simulink model "MADKAL"  (R2015a)
settings: Solver=ode45  StartTime=0.0  StopTime=10.0  RelTol=1e-3
values from neighbouring files (symbols this model uses):
  ba_e = zeros(3,1)    [Parameters.m]
  bb_e = 0    [Parameters.m]
  bg_e = zeros(3,1)    [Parameters.m]
  bm_e = zeros(3,1)    [Parameters.m]
  Ex = zeros(10,1)    [Parameters.m]
  g = 9.81    [Parameters.m]
  g_e = g    (= 9.81)    [Parameters.m]
  G_e = eye(3)    [Parameters.m]
  Ix_e = Ixx    (= 0.034736)    [Parameters.m]
  Iy_e = Iyy    (= 0.034736)    [Parameters.m]
  Iz_e = Izz    (= 0.069472)    [Parameters.m]
  kb_e = 1    [Parameters.m]
  m_e = m    (= 1.478)    [Parameters.m]
  Ma_e = eye(3)    [Parameters.m]
  mag_field = mag / norm(mag)    [Parameters.m]
  mf_e = mf_e /norm(mf_e)    [Parameters.m]
  Mg_e = eye(3)    [Parameters.m]
  P0 = 101325    [Parameters.m]
  P0_e = P0    (= 101325)    [Parameters.m]
  Q_e = 0.005*eye(10)    [Parameters.m]
  R_e = [ 0.0001   0 0 0 0 0 0 0 0 0 ... (first row only)    [Parameters.m]
  Ra = 286.9    [Parameters.m]
  Ra_e = Ra    (= 286.9)    [Parameters.m]
  T0 = 293.15    [Parameters.m]
  T0_e = T0    (= 293.15)    [Parameters.m]
  Ts = 1/200    (= 0.005)    [Parameters.m]
  Varx = 0.001*eye(10)    [Parameters.m]
undefined symbols (not defined in the file or in its folder): freqMadgwick, gain_aa, poles_aa, zeros_aa
libraries: Quadrotor_tools x16, simulink x1, simulink_extras x1
(part 1 of 2)
settings Model: Creator=Mattia  LastModifiedBy=Mattia

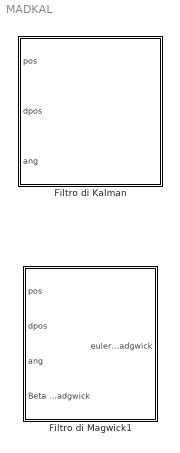
== system MADKAL ==
  Filtro di Kalman : Subsystem
  Filtro di Magwick1 : Subsystem

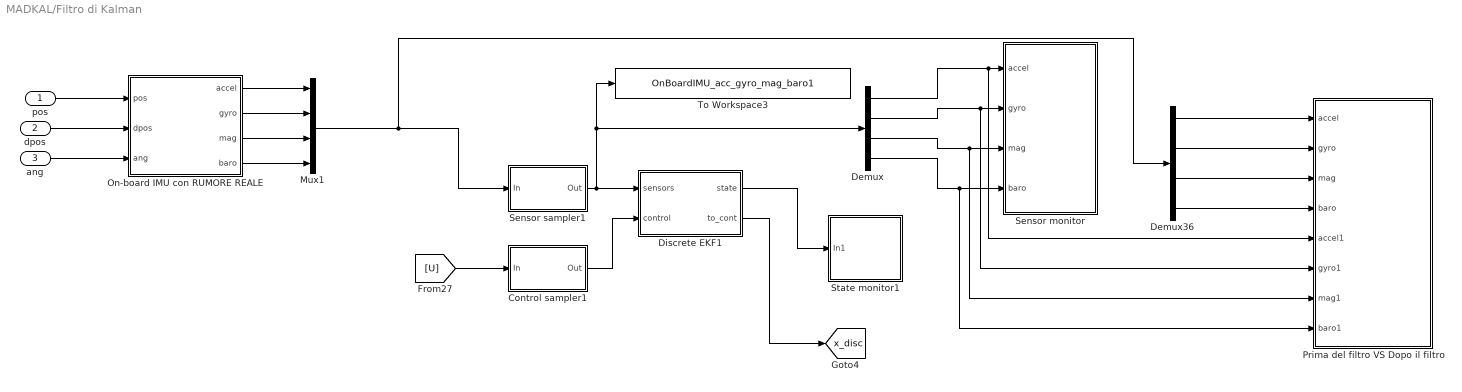
== system MADKAL/Filtro di Kalman ==
  pos : Inport
  dpos : Inport  Port=2
  ang : Inport  Port=3
  Control sampler1 : Subsystem
  Demux : Demux  Outputs=[3 3 3 1]
  Demux36 : Demux  Outputs=[3 3 3 1]
  Discrete EKF1 : Subsystem
  Mux1 : Mux
  On-board IMU con RUMORE REALE : Subsystem
  Prima del filtro VS Dopo il filtro : Subsystem
  Sensor monitor : Subsystem
  Sensor sampler1 : Subsystem
  State monitor1 : Subsystem
  To Workspace3 : ToWorkspace  VariableName=OnBoardIMU_acc_gyro_mag_baro1  SaveFormat=Timeseries  SampleTime=-1
  tag scope: x_disc=global
  wires:
  Demux36/4 -> Prima del filtro VS Dopo il filtro/4(baro)
  Demux36/1 -> Prima del filtro VS Dopo il filtro/1(accel)
  Demux36/2 -> Prima del filtro VS Dopo il filtro/2(gyro)
  Demux36/3 -> Prima del filtro VS Dopo il filtro/3(mag)
  Sensor sampler1/1(Out) -> Discrete EKF1/1(sensors), Demux/1, To Workspace3/1
  [U] -> Control sampler1/1(In)
  Control sampler1/1(Out) -> Discrete EKF1/2(control)
  Demux/1 -> Prima del filtro VS Dopo il filtro/5(accel1), Sensor monitor/1(accel)
  Demux/2 -> Prima del filtro VS Dopo il filtro/6(gyro1), Sensor monitor/2(gyro)
  On-board IMU con RUMORE REALE/1(accel) -> Mux1/1
  Demux/3 -> Prima del filtro VS Dopo il filtro/7(mag1), Sensor monitor/3(mag)
  On-board IMU con RUMORE REALE/4(baro) -> Mux1/4
  On-board IMU con RUMORE REALE/3(mag) -> Mux1/3
  On-board IMU con RUMORE REALE/2(gyro) -> Mux1/2
  Demux/4 -> Prima del filtro VS Dopo il filtro/8(baro1), Sensor monitor/4(baro)
  dpos/1 -> On-board IMU con RUMORE REALE/2(dpos)
  pos/1 -> On-board IMU con RUMORE REALE/1(pos)
  ang/1 -> On-board IMU con RUMORE REALE/3(ang)
  Discrete EKF1/1(state) -> State monitor1/1(In1)
  Discrete EKF1/2("to_cont ") -> [x_disc]
  Mux1/1 -> Sensor sampler1/1(In), Demux36/1

== system MADKAL/Filtro di Magwick1 ==
  pos : Inport
  dpos : Inport  Port=2
  ang : Inport  Port=3
  Beta Madgwick : Inport  Port=4
  Demux11 : Demux  Outputs=[3 3 3 1]
  Madgwickcodice OK2 : Subsystem
  Mux10 : Mux
  On-board IMUcon RUMORE REALE : Subsystem
  Sensor monitor1 : Subsystem
  To Workspace1 : ToWorkspace  VariableName=OnBoardIMU_acc_gyro_mag_baroXX  SaveFormat=Timeseries  SampleTime=-1
  eulero Madgwick : Outport
  wires:
  pos/1 -> On-board IMUcon RUMORE REALE/1(pos)
  ang/1 -> On-board IMUcon RUMORE REALE/3(ang)
  dpos/1 -> On-board IMUcon RUMORE REALE/2(dpos)
  Demux11/4 -> Sensor monitor1/4(baro)
  Demux11/2 -> Sensor monitor1/2(gyro)
  On-board IMUcon RUMORE REALE/1(accel) -> Mux10/1
  Demux11/1 -> Sensor monitor1/1(accel)
  On-board IMUcon RUMORE REALE/3(mag) -> Mux10/3
  On-board IMUcon RUMORE REALE/2(gyro) -> Mux10/2
  Demux11/3 -> Sensor monitor1/3(mag)
  On-board IMUcon RUMORE REALE/4(baro) -> Mux10/4
  Beta Madgwick/1 -> Madgwickcodice OK2/2(Beta Madgwick)
  Madgwickcodice OK2/1(eulerMadgwick) -> eulero Madgwick/1
  Mux10/1 -> To Workspace1/1, Demux11/1, Madgwickcodice OK2/1(In)

== system MADKAL/Filtro di Kalman/Control sampler1 ==
  In : Inport
  Anti-aliasing : Subsystem
  Rate Transition : RateTransition  OutPortSampleTime=Ts
  Out : Outport
  wires:
  Anti-aliasing/1(Out1) -> Rate Transition/1
  In/1 -> Anti-aliasing/1(In1)
  Rate Transition/1 -> Out/1

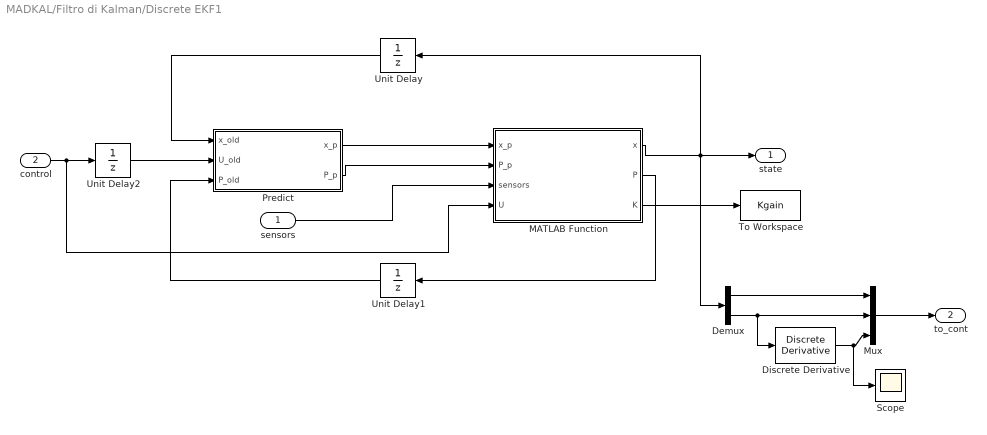
== system MADKAL/Filtro di Kalman/Discrete EKF1 ==
  sensors : Inport
  control : Inport  Port=2
  Demux : Demux  Outputs=[9 1]
  Discrete Derivative : simulink/Discrete/Discrete Derivative  gainval=1.0  ICPrevScaledInput=0.0  InputProcessing=Inherited  OutMin=[]  OutMax=[]  OutDataType=fixdt(1, 16)  OutScaling=2^-10  DoSatur=off
  MATLAB Function : MATLAB Function  TreatAsAtomicUnit=on
  Mux : Mux  Inputs=3
  "Predict " : MATLAB Function  TreatAsAtomicUnit=on
  Scope : Scope
      settings: SaveName=ScopeData20
  To Workspace : ToWorkspace  VariableName=Kgain  SaveFormat=Timeseries  SampleTime=-1
  Unit Delay : UnitDelay  InitialCondition=Ex  SampleTime=Ts
  Unit Delay1 : UnitDelay  InitialCondition=Varx  SampleTime=Ts
  Unit Delay2 : UnitDelay  InitialCondition=[g_e*m_e; 0; 0; 0]  SampleTime=Ts
  state : Outport
  "to_cont " : Outport  Port=2
  wires:
  "Predict "/2(P_p) -> MATLAB Function/2(P_p)
  sensors/1 -> MATLAB Function/3(sensors)
  MATLAB Function/1(x) -> Demux/1, state/1, Unit Delay/1
  Unit Delay/1 -> "Predict "/1(x_old)
  MATLAB Function/2(P) -> Unit Delay1/1
  Unit Delay1/1 -> "Predict "/3(P_old)
  control/1 -> MATLAB Function/4(U), Unit Delay2/1
  Unit Delay2/1 -> "Predict "/2(U_old)
  "Predict "/1(x_p) -> MATLAB Function/1(x_p)
  MATLAB Function/3(K) -> To Workspace/1
  Demux/1 -> Mux/1
  Mux/1 -> "to_cont "/1
  Demux/2 -> Discrete Derivative/1, Mux/2
  Discrete Derivative/1 -> Scope/1, Mux/3

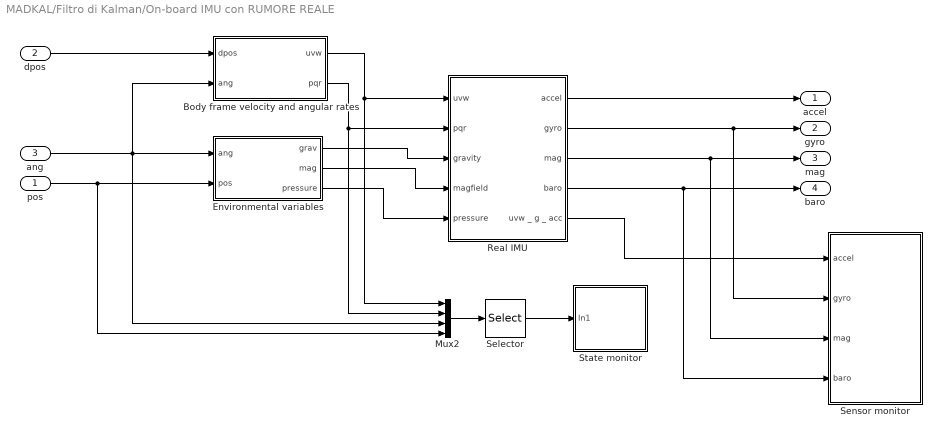
== system MADKAL/Filtro di Kalman/On-board IMU con RUMORE REALE ==
  pos : Inport
  dpos : Inport  Port=2
  ang : Inport  Port=3
  Body frame velocity and angular rates : Subsystem
  Environmental variables : Subsystem
  Mux2 : Mux
  Real IMU : Subsystem
  Selector : Selector  InputPortWidth=12  Indices=[1 2 3 4 5 6 7 8 9 12]
  Sensor monitor : Subsystem
  State monitor : Subsystem
  accel : Outport
  gyro : Outport  Port=2
  mag : Outport  Port=3
  baro : Outport  Port=4
  wires:
  Body frame velocity and angular rates/2(pqr) -> Mux2/2, Real IMU/2(pqr)
  Body frame velocity and angular rates/1(uvw) -> Mux2/1, Real IMU/1(uvw)
  Environmental variables/1(grav) -> Real IMU/3(gravity)
  Environmental variables/2(mag) -> Real IMU/4(magfield)
  Environmental variables/3(pressure) -> Real IMU/5(pressure)
  Mux2/1 -> Selector/1
  Selector/1 -> State monitor/1(In1)
  Real IMU/4(baro) -> Sensor monitor/4(baro), baro/1
  Real IMU/3(mag) -> Sensor monitor/3(mag), mag/1
  Real IMU/2(gyro) -> gyro/1, Sensor monitor/2(gyro)
  Real IMU/1(accel) -> accel/1
  pos/1 -> Mux2/4, Environmental variables/2(pos)
  dpos/1 -> Body frame velocity and angular rates/1(dpos)
  ang/1 -> Body frame velocity and angular rates/2(ang), Mux2/3, Environmental variables/1(ang)
  Real IMU/5(uvw _ g _ acc) -> Sensor monitor/1(accel)

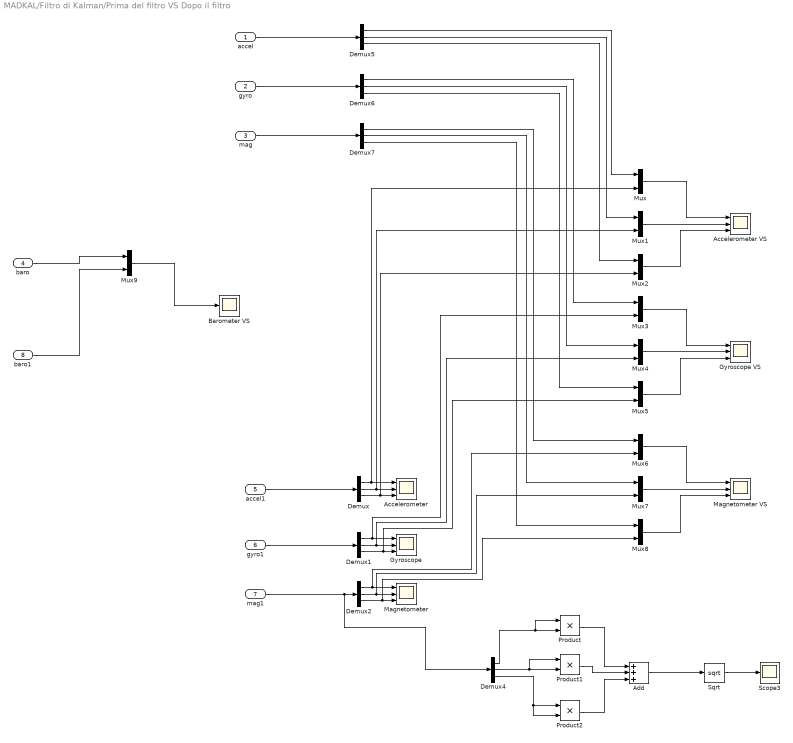
== system MADKAL/Filtro di Kalman/Prima del filtro VS Dopo il filtro ==
  accel : Inport
  gyro : Inport  Port=2
  mag : Inport  Port=3
  baro : Inport  Port=4
  accel1 : Inport  Port=5
  gyro1 : Inport  Port=6
  mag1 : Inport  Port=7
  baro1 : Inport  Port=8
  Accelerometer : Scope  NumInputPorts=3
      settings: YMin=-0.45~-0.4~9.35  YMax=0.4~0.45~10.25  SaveName=ScopeData16
  Accelerometer VS : Scope  NumInputPorts=3
      settings: YMin=-0.45~-0.4~9.35  YMax=0.4~0.45~10.25  SaveName=ScopeData110
  Add : Sum  Inputs=+++
  Barometer VS : Scope
      settings: YMin=-0.45  YMax=0.4  SaveName=ScopeData113
  Demux{,1..2,4..7} (7 alike) : Demux  Outputs=3
  Gyroscope : Scope  NumInputPorts=3
      settings: YMin=-5~-5~-5  YMax=5~5~5  SaveName=ScopeData17
  Gyroscope VS : Scope  NumInputPorts=3
      settings: YMin=-0.45~-0.4~9.35  YMax=0.4~0.45~10.25  SaveName=ScopeData111
  Magnetometer : Scope  NumInputPorts=3
      settings: YMin=-5~-5~-5  YMax=5~5~5  SaveName=ScopeData18
  Magnetometer VS : Scope  NumInputPorts=3
      settings: YMin=-0.45~-0.4~9.35  YMax=0.4~0.45~10.25  SaveName=ScopeData112
  Mux{,1..9} (10 alike) : Mux  Inputs=2
  Product : Product
  Product1 : Product
  Product2 : Product
  Scope3 : Scope
      settings: SaveName=ScopeData103
  Sqrt : Sqrt  SaturateOnIntegerOverflow=on
  wires:
  Demux/3 -> Mux2/2, Accelerometer/3
  Demux/2 -> Mux1/2, Accelerometer/2
  Demux/1 -> Mux/2, Accelerometer/1
  accel1/1 -> Demux/1
  Demux1/3 -> Mux5/2, Gyroscope/3
  Demux1/2 -> Mux4/2, Gyroscope/2
  Demux1/1 -> Mux3/2, Gyroscope/1
  gyro1/1 -> Demux1/1
  Demux2/3 -> Mux8/2, Magnetometer/3
  Demux2/2 -> Mux7/2, Magnetometer/2
  Demux2/1 -> Mux6/2, Magnetometer/1
  mag1/1 -> Demux4/1, Demux2/1
  Demux4/3 -> Product2/2, Product2/1
  Demux4/2 -> Product1/2, Product1/1
  Demux4/1 -> Product/2, Product/1
  Product/1 -> Add/1
  Product1/1 -> Add/2
  Product2/1 -> Add/3
  Add/1 -> Sqrt/1
  Sqrt/1 -> Scope3/1
  Demux5/3 -> Mux2/1
  Demux5/2 -> Mux1/1
  Mux/1 -> Accelerometer VS/1
  Mux1/1 -> Accelerometer VS/2
  Mux2/1 -> Accelerometer VS/3
  Mux3/1 -> Gyroscope VS/1
  Mux4/1 -> Gyroscope VS/2
  Mux5/1 -> Gyroscope VS/3
  Mux6/1 -> Magnetometer VS/1
  Mux7/1 -> Magnetometer VS/2
  Mux8/1 -> Magnetometer VS/3
  Demux5/1 -> Mux/1
  Demux6/1 -> Mux3/1
  Demux6/2 -> Mux4/1
  Demux6/3 -> Mux5/1
  Demux7/1 -> Mux6/1
  Demux7/2 -> Mux7/1
  Demux7/3 -> Mux8/1
  accel/1 -> Demux5/1
  gyro/1 -> Demux6/1
  mag/1 -> Demux7/1
  Mux9/1 -> Barometer VS/1
  baro/1 -> Mux9/1
  baro1/1 -> Mux9/2

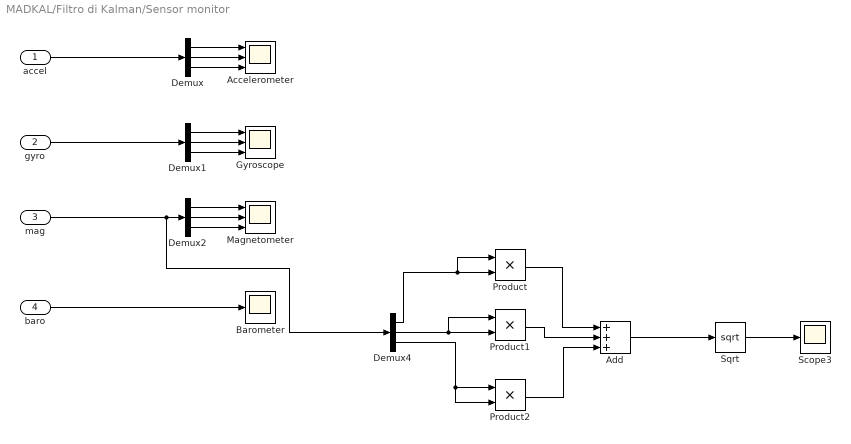
== system MADKAL/Filtro di Kalman/Sensor monitor ==
  accel : Inport
  gyro : Inport  Port=2
  mag : Inport  Port=3
  baro : Inport  Port=4
  Accelerometer : Scope  NumInputPorts=3
      settings: YMin=-0.45~-0.4~9.35  YMax=0.4~0.45~10.25  SaveName=ScopeData16
  Add : Sum  Inputs=+++
  Barometer : Scope
      settings: SaveName=ScopeData19
  Demux{,1..2,4} (4 alike) : Demux  Outputs=3
  Gyroscope : Scope  NumInputPorts=3
      settings: YMin=-5~-5~-5  YMax=5~5~5  SaveName=ScopeData17
  Magnetometer : Scope  NumInputPorts=3
      settings: YMin=-5~-5~-5  YMax=5~5~5  SaveName=ScopeData18
  Product : Product
  Product1 : Product
  Product2 : Product
  Scope3 : Scope
      settings: SaveName=ScopeData103
  Sqrt : Sqrt  SaturateOnIntegerOverflow=on
  wires:
  Demux/3 -> Accelerometer/3
  Demux/2 -> Accelerometer/2
  Demux/1 -> Accelerometer/1
  accel/1 -> Demux/1
  Demux1/3 -> Gyroscope/3
  Demux1/2 -> Gyroscope/2
  Demux1/1 -> Gyroscope/1
  gyro/1 -> Demux1/1
  Demux2/3 -> Magnetometer/3
  Demux2/2 -> Magnetometer/2
  Demux2/1 -> Magnetometer/1
  mag/1 -> Demux4/1, Demux2/1
  baro/1 -> Barometer/1
  Demux4/3 -> Product2/2, Product2/1
  Demux4/2 -> Product1/2, Product1/1
  Demux4/1 -> Product/2, Product/1
  Product/1 -> Add/1
  Product1/1 -> Add/2
  Product2/1 -> Add/3
  Add/1 -> Sqrt/1
  Sqrt/1 -> Scope3/1

== system MADKAL/Filtro di Kalman/Sensor sampler1 ==
  In : Inport
  Anti-aliasing : Subsystem
  Rate Transition : RateTransition  OutPortSampleTime=Ts
  Out : Outport
  wires:
  Rate Transition/1 -> Out/1
  In/1 -> Anti-aliasing/1(In)
  Anti-aliasing/1(Out) -> Rate Transition/1

== system MADKAL/Filtro di Kalman/State monitor1 ==
  In1 : Inport
  Altitude : Scope
      settings: SaveName=ScopeData4
  Angular position : Scope  NumInputPorts=3
      settings: YMin=-5~-5~-5  YMax=5~5~5  SaveName=ScopeData15
  Angular velocity : Scope  NumInputPorts=3
      settings: YMin=-5~-5~-5  YMax=5~5~5  SaveName=ScopeData14
  Demux : Demux  Outputs=[3 3 3 1]
  Demux1 : Demux  Outputs=3
  Demux2 : Demux  Outputs=3
  Demux3 : Demux  Outputs=3
  Linear velocity : Scope  NumInputPorts=3
      settings: YMin=-5~-5~-5  YMax=5~5~5  SaveName=ScopeData13
  To Workspace : ToWorkspace  VariableName=EKFdiscreto_RollPitchYaw  SaveFormat=Timeseries  SampleTime=-1
  tag scope: angKFdisc=global
  wires:
  In1/1 -> Demux/1
  Demux/4 -> Altitude/1
  Demux/1 -> Demux1/1
  Demux1/3 -> Linear velocity/3
  Demux1/2 -> Linear velocity/2
  Demux1/1 -> Linear velocity/1
  Demux/2 -> Demux2/1
  Demux2/3 -> Angular velocity/3
  Demux2/2 -> Angular velocity/2
  Demux2/1 -> Angular velocity/1
  Demux/3 -> [angKFdisc], To Workspace/1, Demux3/1
  Demux3/3 -> Angular position/3
  Demux3/2 -> Angular position/2
  Demux3/1 -> Angular position/1

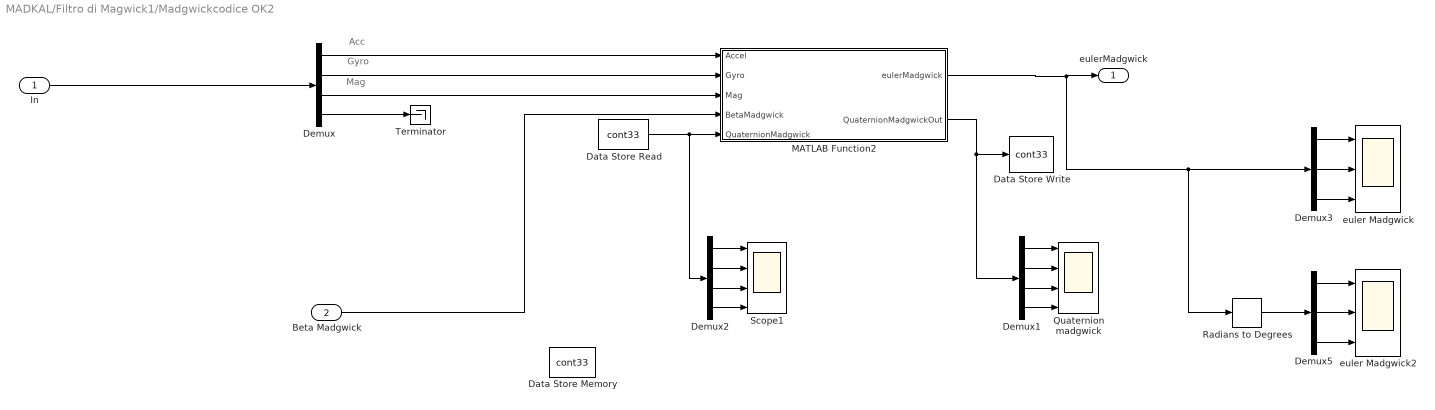
== system MADKAL/Filtro di Magwick1/Madgwickcodice OK2 ==
  note: Mag
  note: Gyro
  note: Acc
  In : Inport
  Beta Madgwick : Inport  Port=2
  Data Store Memory : DataStoreMemory  DataStoreName=cont33  ReadBeforeWriteMsg=warning  WriteAfterWriteMsg=warning  WriteAfterReadMsg=warning  InitialValue=[1 0 0 0]
  Data Store Read : DataStoreRead  DataStoreName=cont33
  Data Store Write : DataStoreWrite  DataStoreName=cont33
  Demux : Demux  Outputs=[3 3 3 1]
  Demux1 : Demux
  Demux2 : Demux
  Demux3 : Demux  Outputs=3
  Demux5 : Demux  Outputs=3
  MATLAB Function2 : MATLAB Function  TreatAsAtomicUnit=on
  Quaternion madgwick : Scope  NumInputPorts=4
      settings: YMin=-5~-5~-5~-5  YMax=5~5~5~5  SaveName=ScopeData89
  Radians to Degrees : simulink_extras/Transformations/Radians to Degrees
  Scope1 : Scope  NumInputPorts=4
      settings: YMin=-5~-5~-5~-5  YMax=5~5~5~5  SaveName=ScopeData90
  Terminator : Terminator
  euler Madgwick : Scope  NumInputPorts=3
      settings: YMin=-5~-5~-5  YMax=5~5~5  SaveName=ScopeData91
  euler Madgwick2 : Scope  NumInputPorts=3
      settings: TimeRange=50  YMin=-5~-5~-5  YMax=5~5~5  SaveName=ScopeData94
  eulerMadgwick : Outport
  wires:
  In/1 -> Demux/1
  Demux/1 -> MATLAB Function2/1(Accel)
  Demux/4 -> Terminator/1
  Demux/3 -> MATLAB Function2/3(Mag)
  Demux/2 -> MATLAB Function2/2(Gyro)
  Data Store Read/1 -> Demux2/1, MATLAB Function2/5(QuaternionMadgwick)
  MATLAB Function2/2(QuaternionMadgwickOut) -> Demux1/1, Data Store Write/1
  Demux1/3 -> Quaternion madgwick/3
  Demux1/4 -> Quaternion madgwick/4
  Demux1/2 -> Quaternion madgwick/2
  Demux1/1 -> Quaternion madgwick/1
  Demux2/3 -> Scope1/3
  Demux2/1 -> Scope1/1
  Demux2/2 -> Scope1/2
  Demux2/4 -> Scope1/4
  Demux3/3 -> euler Madgwick/3
  Demux3/2 -> euler Madgwick/2
  Demux3/1 -> euler Madgwick/1
  Demux5/3 -> euler Madgwick2/3
  Demux5/2 -> euler Madgwick2/2
  Demux5/1 -> euler Madgwick2/1
  Radians to Degrees/1 -> Demux5/1
  Beta Madgwick/1 -> MATLAB Function2/4(BetaMadgwick)
  MATLAB Function2/1(eulerMadgwick) -> Radians to Degrees/1, Demux3/1, eulerMadgwick/1

== system MADKAL/Filtro di Magwick1/On-board IMUcon RUMORE REALE ==
  pos : Inport
  dpos : Inport  Port=2
  ang : Inport  Port=3
  Body frame velocity and angular rates : Subsystem
  Environmental variables : Subsystem
  Mux2 : Mux
  Real IMU : Subsystem
  Selector : Selector  InputPortWidth=12  Indices=[1 2 3 4 5 6 7 8 9 12]
  Sensor monitor : Subsystem
  State monitor : Subsystem
  accel : Outport
  gyro : Outport  Port=2
  mag : Outport  Port=3
  baro : Outport  Port=4
  wires:
  Body frame velocity and angular rates/2(pqr) -> Mux2/2, Real IMU/2(pqr)
  Body frame velocity and angular rates/1(uvw) -> Mux2/1, Real IMU/1(uvw)
  Environmental variables/1(grav) -> Real IMU/3(gravity)
  Environmental variables/2(mag) -> Real IMU/4(magfield)
  Environmental variables/3(pressure) -> Real IMU/5(pressure)
  Mux2/1 -> Selector/1
  Selector/1 -> State monitor/1(In1)
  Real IMU/4(baro) -> Sensor monitor/4(baro), baro/1
  Real IMU/3(mag) -> Sensor monitor/3(mag), mag/1
  Real IMU/2(gyro) -> gyro/1, Sensor monitor/2(gyro)
  Real IMU/1(accel) -> accel/1
  pos/1 -> Mux2/4, Environmental variables/2(pos)
  dpos/1 -> Body frame velocity and angular rates/1(dpos)
  ang/1 -> Body frame velocity and angular rates/2(ang), Mux2/3, Environmental variables/1(ang)
  Real IMU/5(uvw _ g _ acc) -> Sensor monitor/1(accel)

== system MADKAL/Filtro di Magwick1/Sensor monitor1 ==
  accel : Inport
  gyro : Inport  Port=2
  mag : Inport  Port=3
  baro : Inport  Port=4
  Accelerometer : Scope  NumInputPorts=3
      settings: YMin=-5~-5~-5  YMax=5~5~5  SaveName=ScopeData16
  Barometer : Scope
      settings: SaveName=ScopeData19
  Demux : Demux  Outputs=3
  Demux1 : Demux  Outputs=3
  Demux2 : Demux  Outputs=3
  Gyroscope : Scope  NumInputPorts=3
      settings: YMin=-5~-5~-5  YMax=5~5~5  SaveName=ScopeData17
  Magnetometer : Scope  NumInputPorts=3
      settings: YMin=-5~-5~-5  YMax=5~5~5  SaveName=ScopeData18
  wires:
  Demux/3 -> Accelerometer/3
  Demux/2 -> Accelerometer/2
  Demux/1 -> Accelerometer/1
  accel/1 -> Demux/1
  Demux1/3 -> Gyroscope/3
  Demux1/2 -> Gyroscope/2
  Demux1/1 -> Gyroscope/1
  gyro/1 -> Demux1/1
  Demux2/3 -> Magnetometer/3
  Demux2/2 -> Magnetometer/2
  Demux2/1 -> Magnetometer/1
  mag/1 -> Demux2/1
  baro/1 -> Barometer/1

== system MADKAL/Filtro di Kalman/Control sampler1/Anti-aliasing ==
  In1 : Inport
  Bias : Bias  Bias=-g_e*m_e
  Bias1 : Bias  Bias=+g_e*m_e
  Demux : Demux
  Mux : Mux
  Zero-Pole{,1..3} (4 alike) : ZeroPole  Zeros=zeros_aa  Poles=poles_aa  Gain=gain_aa
  Out1 : Outport
  wires:
  In1/1 -> Demux/1
  Mux/1 -> Out1/1
  Zero-Pole3/1 -> Mux/4
  Demux/4 -> Zero-Pole3/1
  Zero-Pole2/1 -> Mux/3
  Demux/3 -> Zero-Pole2/1
  Zero-Pole1/1 -> Mux/2
  Demux/2 -> Zero-Pole1/1
  Bias/1 -> Zero-Pole/1
  Demux/1 -> Bias/1
  Bias1/1 -> Mux/1
  Zero-Pole/1 -> Bias1/1

== system MADKAL/Filtro di Kalman/On-board IMU con RUMORE REALE/Body frame velocity and angular rates ==
  dpos : Inport
  ang : Inport  Port=2
  Earth-to-body frame conversion : Quadrotor_tools/Earth-to-body frame conversion
  Euler to pqr conversion : Quadrotor_tools/Euler to pqr  conversion
  uvw : Outport
  pqr : Outport  Port=2
  wires:
  Earth-to-body frame conversion/1 -> uvw/1
  dpos/1 -> Earth-to-body frame conversion/1
  ang/1 -> Earth-to-body frame conversion/2, Euler to pqr conversion/1
  Euler to pqr conversion/1 -> pqr/1

== system MADKAL/Filtro di Kalman/On-board IMU con RUMORE REALE/Environmental variables ==
  ang : Inport
  pos : Inport  Port=2
  Earth-to-body frame conversion gravity : Quadrotor_tools/Earth-to-body frame conversion
  Earth-to-body frame conversion magnetic : Quadrotor_tools/Earth-to-body frame conversion
  Gravity : Constant  Value=[0 0 -g]
  Hard Iron distortion : Bias  Bias=0.0
  MATLAB Function : MATLAB Function  TreatAsAtomicUnit=on
  Magnetic field : Constant  Value=mag_field  VectorParams1D=off
  Product : Product  Multiplication=Matrix(*)  RndMeth=Zero
  Sea level pressure : Constant  Value=T0
  Soft Iron Distortion : Constant  Value=[1 0 0; 0 1 0; 0 0 1]  VectorParams1D=off
  grav : Outport
  mag : Outport  Port=2
  pressure : Outport  Port=3
  wires:
  Gravity/1 -> Earth-to-body frame conversion gravity/1
  Magnetic field/1 -> Earth-to-body frame conversion magnetic/1
  ang/1 -> Earth-to-body frame conversion magnetic/2, Earth-to-body frame conversion gravity/2
  Earth-to-body frame conversion gravity/1 -> grav/1
  Soft Iron Distortion/1 -> Product/1
  Earth-to-body frame conversion magnetic/1 -> Hard Iron distortion/1
  Product/1 -> mag/1
  Hard Iron distortion/1 -> Product/2
  pos/1 -> MATLAB Function/1(pos)
  Sea level pressure/1 -> MATLAB Function/2(T)
  MATLAB Function/1(P) -> pressure/1

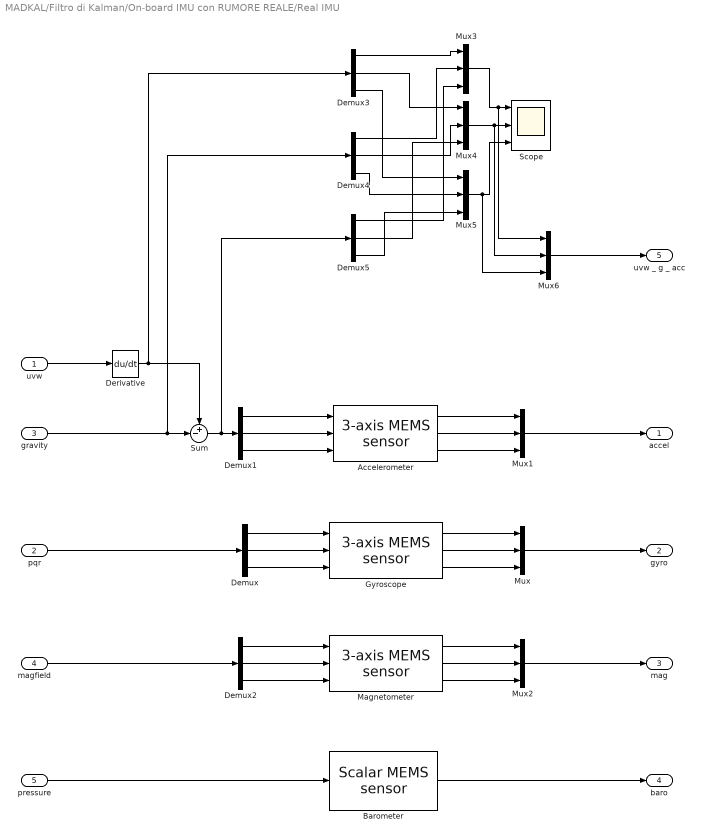
== system MADKAL/Filtro di Kalman/On-board IMU con RUMORE REALE/Real IMU ==
  uvw : Inport
  pqr : Inport  Port=2
  gravity : Inport  Port=3
  magfield : Inport  Port=4
  pressure : Inport  Port=5
  Accelerometer : Quadrotor_tools/3-axis MEMS sensor  biasX=0  biasY=0  biasZ=0  varX=0.0001  varY=0.0001  varZ=0.0001  satUp=20  satLow=-10  delay=0  sampleTime=-1  gainX=1  gainY=1  gainZ=1  gainXY=0  gainXZ=0  gainYX=0  gainYZ=0  gainZX=0  gainZY=0  seedX=73479  seedY=82879  seedZ=96779
  Barometer : Quadrotor_tools/Scalar MEMS sensor  gain=1  bias=0  var=10  seed=1435579  isClipped=on  satUp=130000  satLow=100000  delay=0
  Demux{,1..5} (6 alike) : Demux  Outputs=3
  Derivative : Derivative  CoefficientInTFapproximation=0.001
  Gyroscope : Quadrotor_tools/3-axis MEMS sensor  biasX=0  biasY=0  biasZ=0  varX=0.000008  varY=0.000008  varZ=0.000008  satUp=20  satLow=-20  delay=0  sampleTime=-1  gainX=1  gainY=1  gainZ=1  gainXY=0  gainXZ=0  gainYX=0  gainYZ=0  gainZX=0  gainZY=0  seedX=10179  seedY=52479  seedZ=56579
  Magnetometer : Quadrotor_tools/3-axis MEMS sensor  biasX=0  biasY=0  biasZ=0  varX=0.0001  varY=0.0001  varZ=0.0001  satUp=10  satLow=-10  delay=0  sampleTime=-1  gainX=1  gainY=1  gainZ=1  gainXY=0  gainXZ=0  gainYX=0  gainYZ=0  gainZX=0  gainZY=0  seedX=415179  seedY=456479  seedZ=415379
  Mux{,1..6} (7 alike) : Mux  Inputs=3
  Scope : Scope  NumInputPorts=3
      settings: YMin=-2.5e-06~-4.5e-05~-10  YMax=3.5e-05~2.5e-06~10  SaveName=ScopeData88
  Sum : Sum  Inputs=+-|
  accel : Outport
  gyro : Outport  Port=2
  mag : Outport  Port=3
  baro : Outport  Port=4
  uvw _ g _ acc : Outport  Port=5
  wires:
  pqr/1 -> Demux/1
  Demux/1 -> Gyroscope/1
  Demux/2 -> Gyroscope/2
  Demux/3 -> Gyroscope/3
  Gyroscope/3 -> Mux/3
  Gyroscope/2 -> Mux/2
  Gyroscope/1 -> Mux/1
  uvw/1 -> Derivative/1
  Derivative/1 -> Demux3/1, Sum/1
  Sum/1 -> Demux5/1, Demux1/1
  Demux1/1 -> Accelerometer/1
  Demux1/2 -> Accelerometer/2
  Demux1/3 -> Accelerometer/3
  gravity/1 -> Demux4/1, Sum/2
  Demux2/1 -> Magnetometer/1
  Demux2/2 -> Magnetometer/2
  Demux2/3 -> Magnetometer/3
  Magnetometer/2 -> Mux2/2
  magfield/1 -> Demux2/1
  pressure/1 -> Barometer/1
  Accelerometer/2 -> Mux1/2
  Magnetometer/3 -> Mux2/3
  Magnetometer/1 -> Mux2/1
  Accelerometer/3 -> Mux1/3
  Mux2/1 -> mag/1
  Mux/1 -> gyro/1
  Accelerometer/1 -> Mux1/1
  Mux1/1 -> accel/1
  Barometer/1 -> baro/1
  Mux4/1 -> Mux6/2, Scope/2
  Mux3/1 -> Mux6/1, Scope/1
  Mux5/1 -> Mux6/3, Scope/3
  Demux3/1 -> Mux3/1
  Demux3/2 -> Mux4/1
  Demux3/3 -> Mux5/1
  Demux4/1 -> Mux3/2
  Demux4/2 -> Mux4/2
  Demux4/3 -> Mux5/2
  Demux5/1 -> Mux3/3
  Demux5/2 -> Mux4/3
  Demux5/3 -> Mux5/3
  Mux6/1 -> uvw _ g _ acc/1

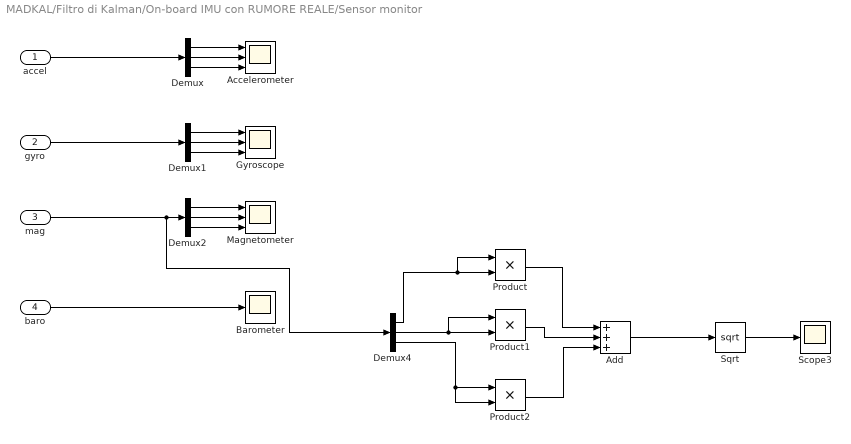
== system MADKAL/Filtro di Kalman/On-board IMU con RUMORE REALE/Sensor monitor ==
  accel : Inport
  gyro : Inport  Port=2
  mag : Inport  Port=3
  baro : Inport  Port=4
  Accelerometer : Scope  NumInputPorts=3
      settings: YMin=-0.45~-0.4~9.35  YMax=0.4~0.45~10.25  SaveName=ScopeData16
  Add : Sum  Inputs=+++
  Barometer : Scope
      settings: SaveName=ScopeData19
  Demux{,1..2,4} (4 alike) : Demux  Outputs=3
  Gyroscope : Scope  NumInputPorts=3
      settings: YMin=-5~-5~-5  YMax=5~5~5  SaveName=ScopeData17
  Magnetometer : Scope  NumInputPorts=3
      settings: YMin=-5~-5~-5  YMax=5~5~5  SaveName=ScopeData18
  Product : Product
  Product1 : Product
  Product2 : Product
  Scope3 : Scope
      settings: SaveName=ScopeData103
  Sqrt : Sqrt  SaturateOnIntegerOverflow=on
  wires:
  Demux/3 -> Accelerometer/3
  Demux/2 -> Accelerometer/2
  Demux/1 -> Accelerometer/1
  accel/1 -> Demux/1
  Demux1/3 -> Gyroscope/3
  Demux1/2 -> Gyroscope/2
  Demux1/1 -> Gyroscope/1
  gyro/1 -> Demux1/1
  Demux2/3 -> Magnetometer/3
  Demux2/2 -> Magnetometer/2
  Demux2/1 -> Magnetometer/1
  mag/1 -> Demux4/1, Demux2/1
  baro/1 -> Barometer/1
  Demux4/3 -> Product2/2, Product2/1
  Demux4/2 -> Product1/2, Product1/1
  Demux4/1 -> Product/2, Product/1
  Product/1 -> Add/1
  Product1/1 -> Add/2
  Product2/1 -> Add/3
  Add/1 -> Sqrt/1
  Sqrt/1 -> Scope3/1

== system MADKAL/Filtro di Kalman/On-board IMU con RUMORE REALE/State monitor ==
  In1 : Inport
  Altitude : Scope
      settings: SaveName=ScopeData4
  Angular position : Scope  NumInputPorts=3
      settings: YMin=-5~-5~-5  YMax=5~5~5  SaveName=ScopeData15
  Angular velocity : Scope  NumInputPorts=3
      settings: YMin=-5~-5~-5  YMax=5~5~5  SaveName=ScopeData14
  Demux : Demux  Outputs=[3 3 3 1]
  Demux1 : Demux  Outputs=3
  Demux2 : Demux  Outputs=3
  Demux3 : Demux  Outputs=3
  Linear velocity : Scope  NumInputPorts=3
      settings: YMin=-5~-5~-5  YMax=5~5~5  SaveName=ScopeData13
  wires:
  In1/1 -> Demux/1
  Demux/4 -> Altitude/1
  Demux/1 -> Demux1/1
  Demux1/3 -> Linear velocity/3
  Demux1/2 -> Linear velocity/2
  Demux1/1 -> Linear velocity/1
  Demux/2 -> Demux2/1
  Demux2/3 -> Angular velocity/3
  Demux2/2 -> Angular velocity/2
  Demux2/1 -> Angular velocity/1
  Demux/3 -> Demux3/1
  Demux3/3 -> Angular position/3
  Demux3/2 -> Angular position/2
  Demux3/1 -> Angular position/1

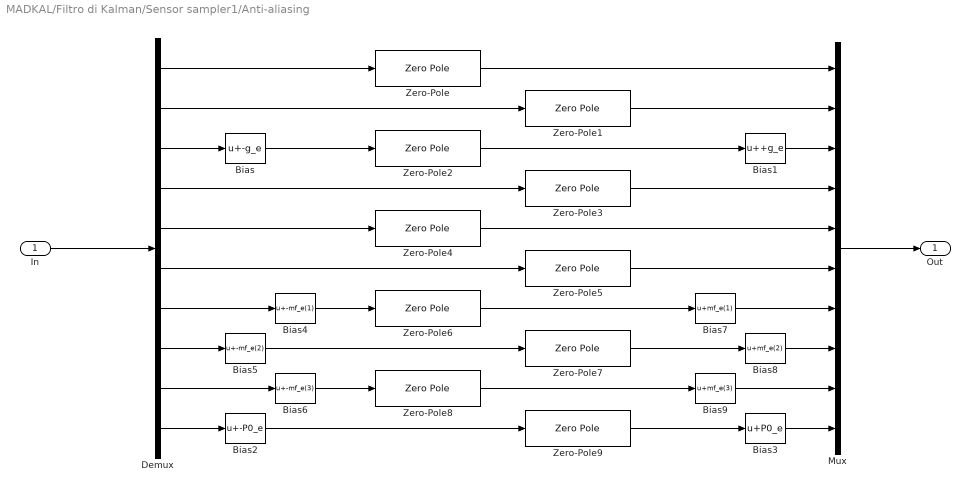
== system MADKAL/Filtro di Kalman/Sensor sampler1/Anti-aliasing ==
  In : Inport
  Bias : Bias  Bias=-g_e
  Bias1 : Bias  Bias=+g_e
  Bias2 : Bias  Bias=-P0_e
  Bias3 : Bias  Bias=P0_e
  Bias4 : Bias  Bias=-mf_e(1)
  Bias5 : Bias  Bias=-mf_e(2)
  Bias6 : Bias  Bias=-mf_e(3)
  Bias7 : Bias  Bias=mf_e(1)
  Bias8 : Bias  Bias=mf_e(2)
  Bias9 : Bias  Bias=mf_e(3)
  Demux : Demux  Outputs=10
  Mux : Mux  Inputs=10
  Zero-Pole{,1..9} (10 alike) : ZeroPole  Zeros=zeros_aa  Poles=poles_aa  Gain=gain_aa
  Out : Outport
  wires:
  In/1 -> Demux/1
  Mux/1 -> Out/1
  Demux/1 -> Zero-Pole/1
  Zero-Pole/1 -> Mux/1
  Demux/2 -> Zero-Pole1/1
  Zero-Pole1/1 -> Mux/2
  Demux/4 -> Zero-Pole3/1
  Zero-Pole3/1 -> Mux/4
  Demux/5 -> Zero-Pole4/1
  Zero-Pole4/1 -> Mux/5
  Demux/9 -> Bias6/1
  Zero-Pole8/1 -> Bias9/1
  Zero-Pole2/1 -> Bias1/1
  Demux/3 -> Bias/1
  Demux/10 -> Bias2/1
  Zero-Pole9/1 -> Bias3/1
  Bias/1 -> Zero-Pole2/1
  Bias1/1 -> Mux/3
  Bias2/1 -> Zero-Pole9/1
  Bias3/1 -> Mux/10
  Bias6/1 -> Zero-Pole8/1
  Bias9/1 -> Mux/9
  Bias8/1 -> Mux/8
  Zero-Pole7/1 -> Bias8/1
  Bias5/1 -> Zero-Pole7/1
  Demux/8 -> Bias5/1
  Bias4/1 -> Zero-Pole6/1
  Demux/7 -> Bias4/1
  Bias7/1 -> Mux/7
  Zero-Pole6/1 -> Bias7/1
  Zero-Pole5/1 -> Mux/6
  Demux/6 -> Zero-Pole5/1

== system MADKAL/Filtro di Magwick1/On-board IMUcon RUMORE REALE/Body frame velocity and angular rates ==
  dpos : Inport
  ang : Inport  Port=2
  Earth-to-body frame conversion : Quadrotor_tools/Earth-to-body frame conversion
  Euler to pqr conversion : Quadrotor_tools/Euler to pqr  conversion
  uvw : Outport
  pqr : Outport  Port=2
  wires:
  Earth-to-body frame conversion/1 -> uvw/1
  dpos/1 -> Earth-to-body frame conversion/1
  ang/1 -> Earth-to-body frame conversion/2, Euler to pqr conversion/1
  Euler to pqr conversion/1 -> pqr/1

== system MADKAL/Filtro di Magwick1/On-board IMUcon RUMORE REALE/Environmental variables ==
  ang : Inport
  pos : Inport  Port=2
  Earth-to-body frame conversion gravity : Quadrotor_tools/Earth-to-body frame conversion
  Earth-to-body frame conversion magnetic : Quadrotor_tools/Earth-to-body frame conversion
  Gravity : Constant  Value=[0 0 -g]
  Hard Iron distortion : Bias  Bias=0.0
  MATLAB Function : MATLAB Function  TreatAsAtomicUnit=on
  Magnetic field : Constant  Value=mag_field  VectorParams1D=off
  Product : Product  Multiplication=Matrix(*)  RndMeth=Zero
  Sea level pressure : Constant  Value=T0
  Soft Iron Distortion : Constant  Value=[1 0 0; 0 1 0; 0 0 1]  VectorParams1D=off
  grav : Outport
  mag : Outport  Port=2
  pressure : Outport  Port=3
  wires:
  Gravity/1 -> Earth-to-body frame conversion gravity/1
  Magnetic field/1 -> Earth-to-body frame conversion magnetic/1
  ang/1 -> Earth-to-body frame conversion magnetic/2, Earth-to-body frame conversion gravity/2
  Earth-to-body frame conversion gravity/1 -> grav/1
  Soft Iron Distortion/1 -> Product/1
  Earth-to-body frame conversion magnetic/1 -> Hard Iron distortion/1
  Product/1 -> mag/1
  Hard Iron distortion/1 -> Product/2
  pos/1 -> MATLAB Function/1(pos)
  Sea level pressure/1 -> MATLAB Function/2(T)
  MATLAB Function/1(P) -> pressure/1

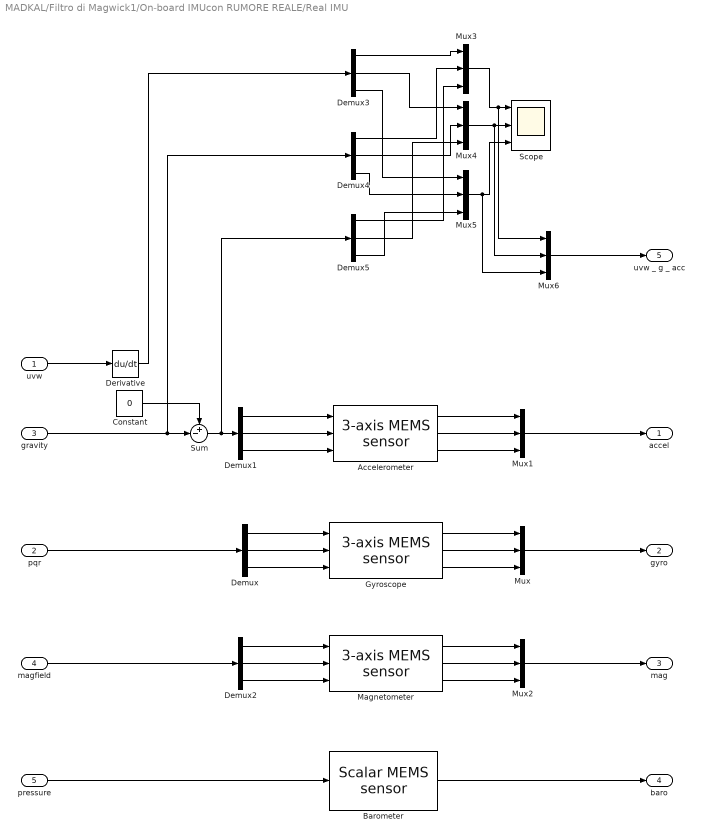
== system MADKAL/Filtro di Magwick1/On-board IMUcon RUMORE REALE/Real IMU ==
  uvw : Inport
  pqr : Inport  Port=2
  gravity : Inport  Port=3
  magfield : Inport  Port=4
  pressure : Inport  Port=5
  Accelerometer : Quadrotor_tools/3-axis MEMS sensor  biasX=0  biasY=0  biasZ=0  varX=0.0001  varY=0.0001  varZ=0.0001  satUp=20  satLow=-10  delay=0  sampleTime=-1  gainX=1  gainY=1  gainZ=1  gainXY=0  gainXZ=0  gainYX=0  gainYZ=0  gainZX=0  gainZY=0  seedX=73479  seedY=82879  seedZ=96779
  Barometer : Quadrotor_tools/Scalar MEMS sensor  gain=1  bias=0  var=10  seed=1435579  isClipped=on  satUp=130000  satLow=100000  delay=0
  Constant : Constant  Value=0
  Demux{,1..5} (6 alike) : Demux  Outputs=3
  Derivative : Derivative  CoefficientInTFapproximation=0.001
  Gyroscope : Quadrotor_tools/3-axis MEMS sensor  biasX=0  biasY=0  biasZ=0  varX=0.000008  varY=0.000008  varZ=0.000008  satUp=20  satLow=-20  delay=0  sampleTime=-1  gainX=1  gainY=1  gainZ=1  gainXY=0  gainXZ=0  gainYX=0  gainYZ=0  gainZX=0  gainZY=0  seedX=10179  seedY=52479  seedZ=56579
  Magnetometer : Quadrotor_tools/3-axis MEMS sensor  biasX=0  biasY=0  biasZ=0  varX=0.0001  varY=0.0001  varZ=0.0001  satUp=10  satLow=-10  delay=0  sampleTime=-1  gainX=1  gainY=1  gainZ=1  gainXY=0  gainXZ=0  gainYX=0  gainYZ=0  gainZX=0  gainZY=0  seedX=415179  seedY=456479  seedZ=415379
  Mux{,1..6} (7 alike) : Mux  Inputs=3
  Scope : Scope  NumInputPorts=3
      settings: YMin=-2.5e-06~-4.5e-05~-10  YMax=3.5e-05~2.5e-06~10  SaveName=ScopeData88
  Sum : Sum  Inputs=+-|
  accel : Outport
  gyro : Outport  Port=2
  mag : Outport  Port=3
  baro : Outport  Port=4
  uvw _ g _ acc : Outport  Port=5
  wires:
  pqr/1 -> Demux/1
  Demux/1 -> Gyroscope/1
  Demux/2 -> Gyroscope/2
  Demux/3 -> Gyroscope/3
  Gyroscope/3 -> Mux/3
  Gyroscope/2 -> Mux/2
  Gyroscope/1 -> Mux/1
  uvw/1 -> Derivative/1
  Derivative/1 -> Demux3/1
  Sum/1 -> Demux5/1, Demux1/1
  Demux1/1 -> Accelerometer/1
  Demux1/2 -> Accelerometer/2
  Demux1/3 -> Accelerometer/3
  gravity/1 -> Demux4/1, Sum/2
  Demux2/1 -> Magnetometer/1
  Demux2/2 -> Magnetometer/2
  Demux2/3 -> Magnetometer/3
  Magnetometer/2 -> Mux2/2
  magfield/1 -> Demux2/1
  pressure/1 -> Barometer/1
  Accelerometer/2 -> Mux1/2
  Magnetometer/3 -> Mux2/3
  Magnetometer/1 -> Mux2/1
  Accelerometer/3 -> Mux1/3
  Mux2/1 -> mag/1
  Mux/1 -> gyro/1
  Accelerometer/1 -> Mux1/1
  Mux1/1 -> accel/1
  Barometer/1 -> baro/1
  Mux4/1 -> Mux6/2, Scope/2
  Mux3/1 -> Mux6/1, Scope/1
  Mux5/1 -> Mux6/3, Scope/3
  Demux3/1 -> Mux3/1
  Demux3/2 -> Mux4/1
  Demux3/3 -> Mux5/1
  Demux4/1 -> Mux3/2
  Demux4/2 -> Mux4/2
  Demux4/3 -> Mux5/2
  Demux5/1 -> Mux3/3
  Demux5/2 -> Mux4/3
  Demux5/3 -> Mux5/3
  Mux6/1 -> uvw _ g _ acc/1
  Constant/1 -> Sum/1

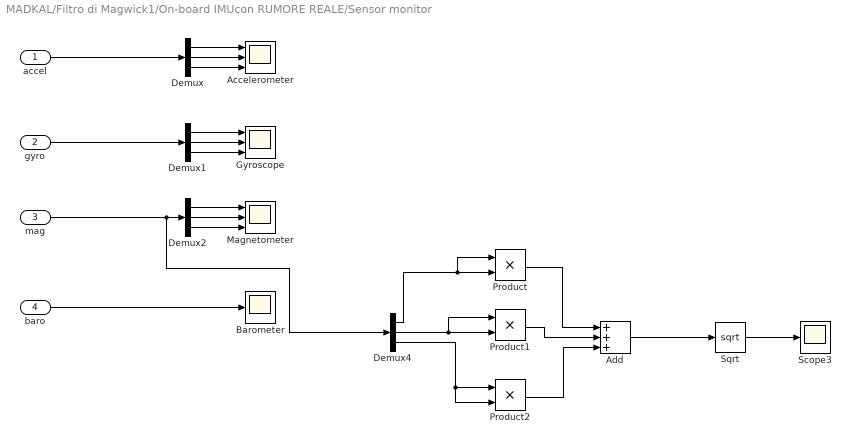
== system MADKAL/Filtro di Magwick1/On-board IMUcon RUMORE REALE/Sensor monitor ==
  accel : Inport
  gyro : Inport  Port=2
  mag : Inport  Port=3
  baro : Inport  Port=4
  Accelerometer : Scope  NumInputPorts=3
      settings: YMin=-0.45~-0.4~9.35  YMax=0.4~0.45~10.25  SaveName=ScopeData16
  Add : Sum  Inputs=+++
  Barometer : Scope
      settings: SaveName=ScopeData19
  Demux{,1..2,4} (4 alike) : Demux  Outputs=3
  Gyroscope : Scope  NumInputPorts=3
      settings: YMin=-5~-5~-5  YMax=5~5~5  SaveName=ScopeData17
  Magnetometer : Scope  NumInputPorts=3
      settings: YMin=-5~-5~-5  YMax=5~5~5  SaveName=ScopeData18
  Product : Product
  Product1 : Product
  Product2 : Product
  Scope3 : Scope
      settings: SaveName=ScopeData103
  Sqrt : Sqrt  SaturateOnIntegerOverflow=on
  wires:
  Demux/3 -> Accelerometer/3
  Demux/2 -> Accelerometer/2
  Demux/1 -> Accelerometer/1
  accel/1 -> Demux/1
  Demux1/3 -> Gyroscope/3
  Demux1/2 -> Gyroscope/2
  Demux1/1 -> Gyroscope/1
  gyro/1 -> Demux1/1
  Demux2/3 -> Magnetometer/3
  Demux2/2 -> Magnetometer/2
  Demux2/1 -> Magnetometer/1
  mag/1 -> Demux4/1, Demux2/1
  baro/1 -> Barometer/1
  Demux4/3 -> Product2/2, Product2/1
  Demux4/2 -> Product1/2, Product1/1
  Demux4/1 -> Product/2, Product/1
  Product/1 -> Add/1
  Product1/1 -> Add/2
  Product2/1 -> Add/3
  Add/1 -> Sqrt/1
  Sqrt/1 -> Scope3/1

== system MADKAL/Filtro di Magwick1/On-board IMUcon RUMORE REALE/State monitor ==
  In1 : Inport
  Altitude : Scope
      settings: SaveName=ScopeData4
  Angular position : Scope  NumInputPorts=3
      settings: YMin=-5~-5~-5  YMax=5~5~5  SaveName=ScopeData15
  Angular velocity : Scope  NumInputPorts=3
      settings: YMin=-5~-5~-5  YMax=5~5~5  SaveName=ScopeData14
  Demux : Demux  Outputs=[3 3 3 1]
  Demux1 : Demux  Outputs=3
  Demux2 : Demux  Outputs=3
  Demux3 : Demux  Outputs=3
  Linear velocity : Scope  NumInputPorts=3
      settings: YMin=-5~-5~-5  YMax=5~5~5  SaveName=ScopeData13
  wires:
  In1/1 -> Demux/1
  Demux/4 -> Altitude/1
  Demux/1 -> Demux1/1
  Demux1/3 -> Linear velocity/3
  Demux1/2 -> Linear velocity/2
  Demux1/1 -> Linear velocity/1
  Demux/2 -> Demux2/1
  Demux2/3 -> Angular velocity/3
  Demux2/2 -> Angular velocity/2
  Demux2/1 -> Angular velocity/1
  Demux/3 -> Demux3/1
  Demux3/3 -> Angular position/3
  Demux3/2 -> Angular position/2
  Demux3/1 -> Angular position/1

== matlab function MADKAL/Filtro di Magwick1/Madgwickcodice OK2/MATLAB Function2 ==
  settings: updateMethod=DISCRETE  sampleTime=1/200
  data: Accel input; eulerMadgwick output; Gyro input; Mag input; freqMadgwick parameter; BetaMadgwick input; QuaternionMadgwick input; g parameter; QuaternionMadgwickOut output
function [eulerMadgwick,QuaternionMadgwickOut]   = fcn(Accel, Gyro, Mag,    freqMadgwick, BetaMadgwick, QuaternionMadgwick,   g)
%#codegen

    
    SampleMadgwick = 1/freqMadgwick;
    eulerMadgwick = ones(1,3);
   
        
%         contatore = contatore +1

   
               
            
       %% Scalatura dati sensori
    
            % Gyroscope
                 Gyroscope = [Gyro(1) Gyro(2) Gyro(3)];       % Gyroscope = [gyroX gyroY gyroZ]
%                  Gyroscope = Gyroscope*17.5*10^-3;  % Deg
                 Gyroscope = Gyroscope*180/pi;
                 
            % Accelerometer
                 Accelerometer = [Accel(1) Accel(2) Accel(3)]/g;   % Accelerometer = [accX accY accZ]
%                  Accelerometer = Accelerometer*10^-3;   % because IMU acceleration is in milli*g
                 Accelerometer = Accelerometer;

%                  % Normalise accelerometer measurement
%                     Acc = Accelerometer;    
%                     AccNorm = Accelerometer / norm(Accelerometer);	% normalise magnitude

            % Magnetometer
                Magnetometer = [Mag(1) Mag(2) Mag(3)];    % Magnetometer = [magX magY magZ]
                 
%                 % MIO - correzione dato magnetometro
%                  Dif = [0.485-cosd(60) -0.015-0.01 -0.875-sind(60)]
%                  Magnetometer = [Mag(1)-Dif(1) Mag(2)-Dif(2) Mag(3)-Dif(3)];    % Magnetometer = [magX magY magZ]
                 % FINE MIO - non ha funzionato

%             % ------------------------------------------------------------------------
%             % Taratura MAGNETOMETRO
%             %          ^^^^^^^^^^^^
% 
%                     % load('Taratura Magnetometro\Taratura_10dic_Sera.mat');    Spostata sopra per velocizzare
% 
%                      xx=MagnetometerRead(1,1)-M_OSx;
%                      yy=MagnetometerRead(1,2)-M_OSy;
%                      zz=MagnetometerRead(1,3)-M_OSz;
% 
%                      xxx=xx./M_SCx;
%                      yyy=yy./M_SCy;
%                      zzz=zz./M_SCz;
% 
%                      MagnetometerTar = [xxx yyy zzz];
%                      
%                      Magnetometer = MagnetometerTar;
                     
                   
                   
                   
      %% Process sensor data through algorithm
            
            % AHRS.Update(Gyroscope*(pi/180), Accelerometer, Magnetometer);	% gyroscope units must be radians
            %   AHRS.UpdateIMU(Gyroscope* (pi/180), Accelerometer);                % giorscopio + accelerometro
           
            Gyroscope = Gyroscope*(pi/180);
            
            % qMadgwick = QuaternionMadgwick; % short name local variable for readability % non gli piace
            qMadgwick = [QuaternionMadgwick(1) QuaternionMadgwick(2) QuaternionMadgwick(3) QuaternionMadgwick(4)];
            
            % Normalise accelerometer measurement
%             if(norm(Accelerometer) == 0), return; end	% handle NaN
            Accelerometer = Accelerometer / norm(Accelerometer);	% normalise magnitude

            % Normalise magnetometer measurement
%             if(norm(Magnetometer) == 0), return; end	% handle NaN
            Magnetometer = Magnetometer / norm(Magnetometer);	% normalise magnitude

            % Reference direction of Earth's magnetic feild
            % hMadgwick = quaternProd(qMadgwick, quaternProd([0 Magnetometer], quaternConj(qMadgwick)));
                    % MIO
                    %QUATERNConj Converts a quaternion to its conjugate
                    qConjqMadgwick = [qMadgwick(1) -qMadgwick(2) -qMadgwick(3) -qMadgwick(4)];
                    
                    qMag = [0 Magnetometer];
                    quaternProdMag = zeros(1,4);
                        %QUATERNPROD Calculates the quaternion product
                        quaternProdMag(1) = qMag(1).*qConjqMadgwick(1)-qMag(2).*qConjqMadgwick(2)-qMag(3).*qConjqMadgwick(3)-qMag(4).*qConjqMadgwick(4);
                        quaternProdMag(2) = qMag(1).*qConjqMadgwick(2)+qMag(2).*qConjqMadgwick(1)+qMag(3).*qConjqMadgwick(4)-qMag(4).*qConjqMadgwick(3);
                        quaternProdMag(3) = qMag(1).*qConjqMadgwick(3)-qMag(2).*qConjqMadgwick(4)+qMag(3).*qConjqMadgwick(1)+qMag(4).*qConjqMadgwick(2);
                        quaternProdMag(4) = qMag(1).*qConjqMadgwick(4)+qMag(2).*qConjqMadgwick(3)-qMag(3).*qConjqMadgwick(2)+qMag(4).*qConjqMadgwick(1);
                    
                    hMadgwick = zeros(1,4);
                        %QUATERNPROD Calculates the quaternion product
                        hMadgwick(1) = qMadgwick(1).*quaternProdMag(1)-qMadgwick(2).*quaternProdMag(2)-qMadgwick(3).*quaternProdMag(3)-qMadgwick(4).*quaternProdMag(4);
                        hMadgwick(2) = qMadgwick(1).*quaternProdMag(2)+qMadgwick(2).*quaternProdMag(1)+qMadgwick(3).*quaternProdMag(4)-qMadgwick(4).*quaternProdMag(3);
                        hMadgwick(3) = qMadgwick(1).*quaternProdMag(3)-qMadgwick(2).*quaternProdMag(4)+qMadgwick(3).*quaternProdMag(1)+qMadgwick(4).*quaternProdMag(2);
                        hMadgwick(4) = qMadgwick(1).*quaternProdMag(4)+qMadgwick(2).*quaternProdMag(3)-qMadgwick(3).*quaternProdMag(2)+qMadgwick(4).*quaternProdMag(1);
                    % fine MIO
                        
            bMadgwick = [0 norm([hMadgwick(2) hMadgwick(3)]) 0 hMadgwick(4)];

            % Gradient decent algorithm corrective step
            FMadgwick = [2*(qMadgwick(2)*qMadgwick(4) - qMadgwick(1)*qMadgwick(3)) - Accelerometer(1)
                2*(qMadgwick(1)*qMadgwick(2) + qMadgwick(3)*qMadgwick(4)) - Accelerometer(2)
                2*(0.5 - qMadgwick(2)^2 - qMadgwick(3)^2) - Accelerometer(3)
                2*bMadgwick(2)*(0.5 - qMadgwick(3)^2 - qMadgwick(4)^2) + 2*bMadgwick(4)*(qMadgwick(2)*qMadgwick(4) - qMadgwick(1)*qMadgwick(3)) - Magnetometer(1)
                2*bMadgwick(2)*(qMadgwick(2)*qMadgwick(3) - qMadgwick(1)*qMadgwick(4)) + 2*bMadgwick(4)*(qMadgwick(1)*qMadgwick(2) + qMadgwick(3)*qMadgwick(4)) - Magnetometer(2)
                2*bMadgwick(2)*(qMadgwick(1)*qMadgwick(3) + qMadgwick(2)*qMadgwick(4)) + 2*bMadgwick(4)*(0.5 - qMadgwick(2)^2 - qMadgwick(3)^2) - Magnetometer(3)];
            JMadgwick = [-2*qMadgwick(3),                 	2*qMadgwick(4),                    -2*qMadgwick(1),                         2*qMadgwick(2)
                2*qMadgwick(2),                 	2*qMadgwick(1),                    	2*qMadgwick(4),                         2*qMadgwick(3)
                0,                         -4*qMadgwick(2),                    -4*qMadgwick(3),                         0
                -2*bMadgwick(4)*qMadgwick(3),               2*bMadgwick(4)*qMadgwick(4),               -4*bMadgwick(2)*qMadgwick(3)-2*bMadgwick(4)*qMadgwick(1),       -4*bMadgwick(2)*qMadgwick(4)+2*bMadgwick(4)*qMadgwick(2)
                -2*bMadgwick(2)*qMadgwick(4)+2*bMadgwick(4)*qMadgwick(2),	2*bMadgwick(2)*qMadgwick(3)+2*bMadgwick(4)*qMadgwick(1),	2*bMadgwick(2)*qMadgwick(2)+2*bMadgwick(4)*qMadgwick(4),       -2*bMadgwick(2)*qMadgwick(1)+2*bMadgwick(4)*qMadgwick(3)
                2*bMadgwick(2)*qMadgwick(3),                2*bMadgwick(2)*qMadgwick(4)-4*bMadgwick(4)*qMadgwick(2),	2*bMadgwick(2)*qMadgwick(1)-4*bMadgwick(4)*qMadgwick(3),        2*bMadgwick(2)*qMadgwick(2)];
            stepMadgwick = (JMadgwick'*FMadgwick);
            stepMadgwick = stepMadgwick / norm(stepMadgwick);	% normalise step magnitude

            % Compute rate of change of quaternion
            % qMadgwickDot = 0.5 * quaternProd(qMadgwick, [0 Gyroscope(1) Gyroscope(2) Gyroscope(3)]) - BetaMadgwick * stepMadgwick';
                    % MIO
                    qGyro = [0 Gyroscope(1) Gyroscope(2) Gyroscope(3)];
                    quaternProdGyro = zeros(1,4);
                    %QUATERNPROD Calculates the quaternion product
                        quaternProdGyro(1) = qMadgwick(1).*qGyro(1)-qMadgwick(2).*qGyro(2)-qMadgwick(3).*qGyro(3)-qMadgwick(4).*qGyro(4);
                        quaternProdGyro(2) = qMadgwick(1).*qGyro(2)+qMadgwick(2).*qGyro(1)+qMadgwick(3).*qGyro(4)-qMadgwick(4).*qGyro(3);
                        quaternProdGyro(3) = qMadgwick(1).*qGyro(3)-qMadgwick(2).*qGyro(4)+qMadgwick(3).*qGyro(1)+qMadgwick(4).*qGyro(2);
                        quaternProdGyro(4) = qMadgwick(1).*qGyro(4)+qMadgwick(2).*qGyro(3)-qMadgwick(3).*qGyro(2)+qMadgwick(4).*qGyro(1);
                    
                    qMadgwickDot = zeros(1,4);    
                    qMadgwickDot = 0.5.* quaternProdGyro - BetaMadgwick.* stepMadgwick';      % non gli piace
                                        
                    % Fine MIO
                    
            % Integrate to yield quaternion
            qMadgwick = qMadgwick + qMadgwickDot * SampleMadgwick;
            QuaternionMadgwick = qMadgwick / norm(qMadgwick); % normalise quaternion
            
            
            
            
        % Convert algorithm output (quaternion) to rotation matrix
        %    RMadgwick(:,:) = quatern2rotMat(QuaternionMadgwick)';     % transpose because ahrs provides Earth relative to sensor
                 % MIO
                 RMadgwick = zeros(3,3); % rotation matrix describing sensor relative to Earth
                        RMadgwick(1,1,:) = 2.*qMadgwick(1).^2-1+2.*qMadgwick(2).^2;
                        RMadgwick(1,2,:) = 2.*(qMadgwick(2).*qMadgwick(3)+qMadgwick(1).*qMadgwick(4));
                        RMadgwick(1,3,:) = 2.*(qMadgwick(2).*qMadgwick(4)-qMadgwick(1).*qMadgwick(3));
                        RMadgwick(2,1,:) = 2.*(qMadgwick(2).*qMadgwick(3)-qMadgwick(1).*qMadgwick(4));
                        RMadgwick(2,2,:) = 2.*qMadgwick(1).^2-1+2.*qMadgwick(3).^2;
                        RMadgwick(2,3,:) = 2.*(qMadgwick(3).*qMadgwick(4)+qMadgwick(1).*qMadgwick(2));
                        RMadgwick(3,1,:) = 2.*(qMadgwick(2).*qMadgwick(4)+qMadgwick(1).*qMadgwick(3));
                        RMadgwick(3,2,:) = 2.*(qMadgwick(3).*qMadgwick(4)-qMadgwick(1).*qMadgwick(2));
                        RMadgwick(3,3,:) = 2.*qMadgwick(1).^2-1+2.*qMadgwick(4).^2;
                RMadgwick = RMadgwick';
                % Fine MIO
        
        % Convert algorithm output (quaternion) to Euler angles (Roll, Pitch, Yaw)
            % The first and third Euler angles in the sequence (phi and psi) become
            % unreliable when the middle angles of the sequence (theta) approaches ±90
            % degrees. This problem commonly referred to as Gimbal Lock.
            % See: http://en.wikipedia.org/wiki/Gimbal_lock
            
            % eulerMadgwick = quatern2euler(quaternConj(QuaternionMadgwick)) * (180/pi);	% use conjugate for sensor frame relative to Earth and convert to degrees.
                % MIO
                quaternConjQuaternionMadgwick = [QuaternionMadgwick(1) -QuaternionMadgwick(2) -QuaternionMadgwick(3) -QuaternionMadgwick(4)];
                RPerEulero = zeros(3,3);
                    RPerEulero(1,1) = 2.*quaternConjQuaternionMadgwick(1).^2-1+2.*quaternConjQuaternionMadgwick(2).^2;
                    RPerEulero(2,1) = 2.*(quaternConjQuaternionMadgwick(2).*quaternConjQuaternionMadgwick(3)-quaternConjQuaternionMadgwick(1).*quaternConjQuaternionMadgwick(4));
                    RPerEulero(3,1) = 2.*(quaternConjQuaternionMadgwick(2).*quaternConjQuaternionMadgwick(4)+quaternConjQuaternionMadgwick(1).*quaternConjQuaternionMadgwick(3));
                    RPerEulero(3,2) = 2.*(quaternConjQuaternionMadgwick(3).*quaternConjQuaternionMadgwick(4)-quaternConjQuaternionMadgwick(1).*quaternConjQuaternionMadgwick(2));
                    RPerEulero(3,3) = 2.*quaternConjQuaternionMadgwick(1).^2-1+2.*quaternConjQuaternionMadgwick(4).^2;
                
                 phi = atan2(RPerEulero(3,2), RPerEulero(3,3) );
                 theta = -atan(RPerEulero(3,1) ./ sqrt(1-RPerEulero(3,1).^2) );
                 psi = atan2(RPerEulero(2,1), RPerEulero(1,1) );

                 % eulerMadgwick = [phi' theta' psi'];
                 eulerMadgwick = [phi theta psi];  % modifica improvvisata MIA
                 % fine MIO
                 
            QuaternionMadgwickOut = QuaternionMadgwick;

== matlab function MADKAL/Filtro di Kalman/On-board IMU con RUMORE REALE/Environmental variables/MATLAB Function ==
  data P0 settings: description=Atmosferic pressure at sea level.
  data T settings: description=Air temperature.
  data Ra settings: description=Air gas constant (depends upon the humidity).
  data g settings: description=Gravitational acceleration.
  data: pos input; P output; P0 parameter; T input; Ra parameter; g parameter
function P = pressure_altitude(pos, P0, T, Ra, g)
%#codegen
% ----------------------------------------------------
% This function calculates the value of the 
% atmospheric pressure given the altitude and 
% the temperature.
% The pressure at sea level P0 is assumed to be a
% constant parameter.
% ----------------------------------------------------

% Extract the altitude from the position vector.
z = pos(3);

P = P0*exp(-(g*z)/(T*Ra));

== matlab function MADKAL/Filtro di Magwick1/On-board IMUcon RUMORE REALE/Environmental variables/MATLAB Function ==
  data P0 settings: description=Atmosferic pressure at sea level.
  data T settings: description=Air temperature.
  data Ra settings: description=Air gas constant (depends upon the humidity).
  data g settings: description=Gravitational acceleration.
  data: pos input; P output; P0 parameter; T input; Ra parameter; g parameter
function P = pressure_altitude(pos, P0, T, Ra, g)
%#codegen
% ----------------------------------------------------
% This function calculates the value of the 
% atmospheric pressure given the altitude and 
% the temperature.
% The pressure at sea level P0 is assumed to be a
% constant parameter.
% ----------------------------------------------------

% Extract the altitude from the position vector.
z = pos(3);

P = P0*exp(-(g*z)/(T*Ra));
